simulink model "Reference_controller"  (R2022b)
settings: Solver=FixedStepAuto  StartTime=0.0  StopTime=600*24  FixedStep=1  RelTol=1e-3
undefined symbols (not defined in the file): c
settings Model: Creator=is123  LastModifiedBy=is123
settings OptimizationCC: ReuseModelBlockBuffer=on

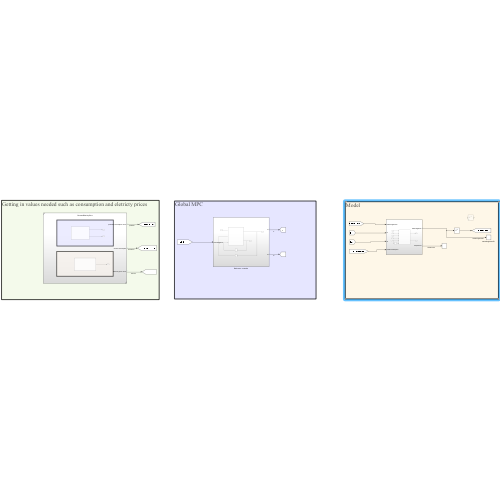
[thumbnail: Simulink's stored preview of the top-level diagram]
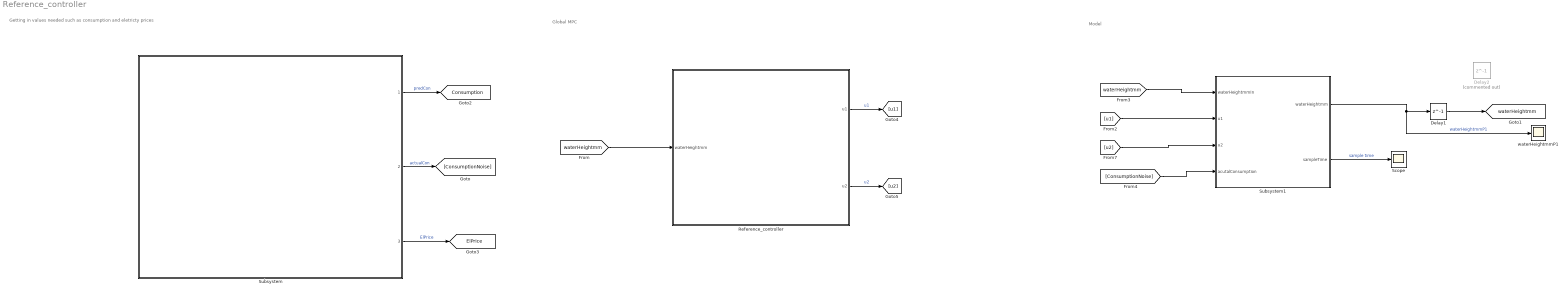
== system Reference_controller ==
  note: Getting in values needed such as consumption and eletricty prices
  note: Global MPC
  note: Model
  Delay1 : Delay  DelayLength=1  InitialCondition=c.V/c.At*1e3
  Delay2 : Delay  Commented=on  DelayLength=1  InitialCondition=534
  Reference_controller : Subsystem
  Scope : Scope
  Subsystem : Subsystem  ReferencedSubsystem=DemandEletricityPrice
  Subsystem1 : Subsystem
  waterHeightmmP1 : Scope
  tag scope: Consumption=global, ElPrice=global, waterHeightmm=global
  wires:
  Subsystem1/1(waterHeightmm) -> waterHeightmmP1/1, Delay1/1  "waterHeightmmP1"
  [waterHeightmm] -> Subsystem1/1(waterHeightmmIn)
  [u1] -> Subsystem1/2(u1)
  [ConsumptionNoise] -> Subsystem1/4(acutalConsumption)
  Subsystem/2 -> [ConsumptionNoise]  "actualCon"
  Subsystem/1 -> [Consumption]  "predCon"
  Subsystem/3 -> [ElPrice]  "ElPrice"
  [u2] -> Subsystem1/3(u2)
  Delay1/1 -> [waterHeightmm]
  Reference_controller/1(u1) -> [u1]  "u1"
  Reference_controller/2(u2) -> [u2]  "u2"
  [waterHeightmm] -> Reference_controller/1(waterHeightmm)
  Subsystem1/2(sampleTime) -> Scope/1  "sample time"

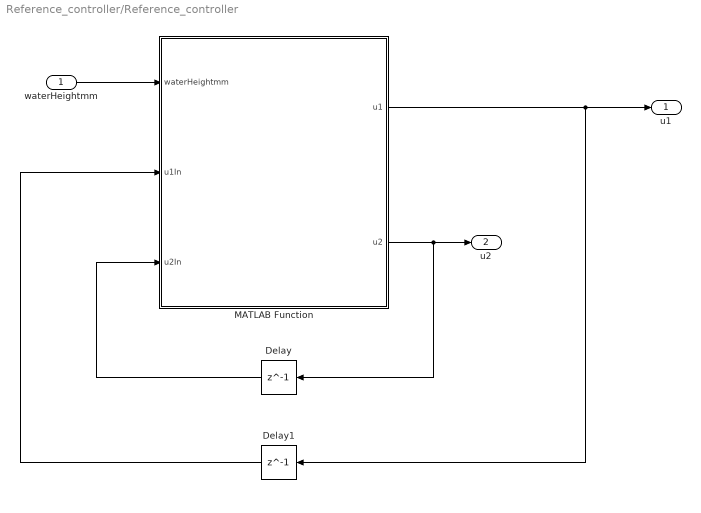
== system Reference_controller/Reference_controller ==
  waterHeightmm : Inport
  Delay : Delay  DelayLength=1  InitialCondition=0
  Delay1 : Delay  DelayLength=1  InitialCondition=0
  MATLAB Function : MATLAB Function  TreatAsAtomicUnit=on
  u1 : Outport
  u2 : Outport  Port=2
  wires:
  MATLAB Function/2(u2) -> Delay/1, u2/1
  MATLAB Function/1(u1) -> Delay1/1, u1/1
  waterHeightmm/1 -> MATLAB Function/1(waterHeightmm)
  Delay/1 -> MATLAB Function/3(u2In)
  Delay1/1 -> MATLAB Function/2(u1In)

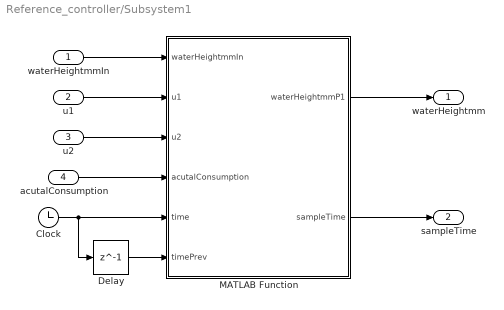
== system Reference_controller/Subsystem1 ==
  waterHeightmmIn : Inport
  u1 : Inport  Port=2
  u2 : Inport  Port=3
  acutalConsumption : Inport  Port=4
  Clock : Clock
  Delay : Delay  DelayLength=1  InitialCondition=0
  MATLAB Function : MATLAB Function  TreatAsAtomicUnit=on
  waterHeightmm : Outport
  sampleTime : Outport  Port=2
  wires:
  waterHeightmmIn/1 -> MATLAB Function/1(waterHeightmmIn)
  MATLAB Function/1(waterHeightmmP1) -> waterHeightmm/1
  u1/1 -> MATLAB Function/2(u1)
  u2/1 -> MATLAB Function/3(u2)
  acutalConsumption/1 -> MATLAB Function/4(acutalConsumption)
  Clock/1 -> Delay/1, MATLAB Function/5(time)
  Delay/1 -> MATLAB Function/6(timePrev)
  MATLAB Function/2(sampleTime) -> sampleTime/1

== matlab function Reference_controller/Subsystem1/MATLAB Function ==
  data: waterHeightmmIn input; waterHeightmmP1 output; u1 input; u2 input; acutalConsumption input; time input; timePrev input; sampleTime output
function [waterHeightmmP1,sampleTime] = fcn(waterHeightmmIn, u1, u2, acutalConsumption,time,timePrev)
c=scaled_standard_constants;
%Getting sample time:
sampleTime= time-timePrev;
c.ts = sampleTime;
d=acutalConsumption;

%Waiting 10 minuts to allow the physical system to start
if time <600 
    waterHeightmmP1=waterHeightmmIn; 
else 
%Setting the output to zero becuase it is needed
waterHeightmmP1=zeros(1,1);

%Collecting the used mass flows into a vector 
u=[u1;u2];

%Determine the water volume instead of water height 
V=waterHeightmmIn/1e3*c.At;

%% Define the state space matrixs (from the report) 
A=1; 
Bu=ones(1,c.Nu)*c.ts/3600; 
Bd=ones(1,c.Nd)*c.ts/3600;

%% Determine the next water volume:  
Vp1=A*V+Bu*u(1:c.Nu,1)-Bd*d(1,1);

%Determine water height instead of water volume: 
waterHeightmmP1=Vp1/c.At*1e3; 
end

== matlab function Reference_controller/MATLAB Function ==
  data: waterHeightmm input; u1 output; u1In input; u2In input; u2 output
function [u1,u2] = fcn(waterHeightmm,u1In,u2In)
c=scaled_standard_constants;

waterHeightmin=c.Vmin/c.At*1000;

waterHeightmax=c.Vmax/c.At*1000; 


if waterHeightmm <= waterHeightmin && u1In==0 && u2In==0 
%     u1=c.umax1;
%     u2=c.umax2; 
    u1=0.2;
    u2=0.2; 
% elseif waterHeightmm < waterHeightmax && u1In==c.umax1 && u2In==c.umax2 
%     u1=c.umax1;
%     u2=c.umax2; 
elseif waterHeightmm > waterHeightmax && u1In==0.2 && u2In==0.2 
    %elseif waterHeightmm > waterHeightmax && u1In==c.umax1 && u2In==c.umax2 
    u1=0; 
    u2=0;
else 
    u1=u1In; 
    u2=u2In;
end
